simulink model "prob2_sim"  (R2013a)
settings: Solver=ode45  StartTime=0.0  StopTime=10.0  RelTol=1e-3
libraries: fl_lib x13, nesl_utility x7
settings Model: Creator=Suddenlink  LastModifiedBy=Suddenlink

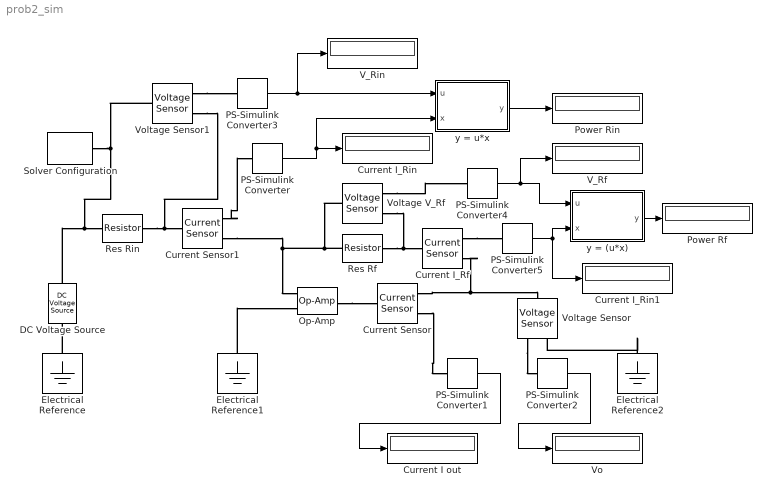
== system prob2_sim ==
  Current I out : Display
  Current I_Rf : fl_lib/Electrical/Electrical Sensors/Current Sensor  i1_Log=off  v1_Log=off  LocalVarNames=|i1|v1  LocalVarDescs=|i1|v1  LocalVarLogging=[0 0]
  Current I_Rin : Display
  Current I_Rin1 : Display
  Current Sensor : fl_lib/Electrical/Electrical Sensors/Current Sensor  i1_Log=off  v1_Log=off  LocalVarNames=|i1|v1  LocalVarDescs=|i1|v1  LocalVarLogging=[0 0]
  Current Sensor1 : fl_lib/Electrical/Electrical Sensors/Current Sensor  i1_Log=off  v1_Log=off  LocalVarNames=|i1|v1  LocalVarDescs=|i1|v1  LocalVarLogging=[0 0]
  DC Voltage Source : fl_lib/Electrical/Electrical Sources/DC Voltage Source  v0=5 V  i_Log=off  v_Log=off  LocalVarNames=|i|v  LocalVarDescs=|i|v  LocalVarLogging=[0 0]
  Electrical Reference : fl_lib/Electrical/Electrical Elements/Electrical Reference  i_Log=off  LocalVarNames=|i  LocalVarDescs=|i  LocalVarLogging=0
  Electrical Reference1 : fl_lib/Electrical/Electrical Elements/Electrical Reference  i_Log=off  LocalVarNames=|i  LocalVarDescs=|i  LocalVarLogging=0
  Electrical Reference2 : fl_lib/Electrical/Electrical Elements/Electrical Reference  i_Log=off  LocalVarNames=|i  LocalVarDescs=|i  LocalVarLogging=0
  Op-Amp : fl_lib/Electrical/Electrical Elements/Op-Amp  i1_Log=off  v1_Log=off  outI_Log=off  LocalVarNames=|i1|v1|outI  LocalVarDescs=|i1|v1|outI  LocalVarLogging=[0 0 0]
  PS-Simulink Converter{,1..5} (6 alike) : nesl_utility/PS-Simulink Converter  PhysicalDomain=network_engine_domain  SubClassName=ps_output  LeftPortType=input  RightPortType=output  PseudoPeriodic=off  Frequencies=[]  Unit=1  AffineConversion=off
  Power Rf : Display
  Power Rin : Display
  Res Rf : fl_lib/Electrical/Electrical Elements/Resistor  R=10000 Ohm  i_Log=off  v_Log=off  LocalVarNames=|i|v  LocalVarDescs=|i|v  LocalVarLogging=[0 0]
  "Res Rin " : fl_lib/Electrical/Electrical Elements/Resistor  R=1000 Ohm  i_Log=off  v_Log=off  LocalVarNames=|i|v  LocalVarDescs=|i|v  LocalVarLogging=[0 0]
  Solver Configuration : nesl_utility/Solver Configuration  PhysicalDomain=network_engine_domain  SubClassName=solver  LeftPortType=input  RightPortType=generic  Accelerate=off  Tones=[]  Harmonics=[]  SimulateNoise=off  Profile=off  UseLocalSampling=off  EnableSwitchedLinearOptims=on  FrequencyDomain=off  UseCCode=off  UseNewInitialization=off  DoDC=off  ResidualTolerance=1e-09  UseLocalSolver=off  LocalSolverChoice=NE_BACKWARD_EULER_ADVANCER  LocalSolverSampleTime=0.001  DoFixedCost=off  MaxNonlinIter=3  MaxModeIter=2  LinearAlgebra=Sparse  DelaysMemoryBudget=1024
  V_Rf : Display
  V_Rin : Display
  Vo : Display
  Voltage Sensor : fl_lib/Electrical/Electrical Sensors/Voltage Sensor  i1_Log=off  v1_Log=off  LocalVarNames=|i1|v1  LocalVarDescs=|i1|v1  LocalVarLogging=[0 0]
  Voltage Sensor1 : fl_lib/Electrical/Electrical Sensors/Voltage Sensor  i1_Log=off  v1_Log=off  LocalVarNames=|i1|v1  LocalVarDescs=|i1|v1  LocalVarLogging=[0 0]
  Voltage V_Rf : fl_lib/Electrical/Electrical Sensors/Voltage Sensor  i1_Log=off  v1_Log=off  LocalVarNames=|i1|v1  LocalVarDescs=|i1|v1  LocalVarLogging=[0 0]
  y = (u*x) : MATLAB Function  TreatAsAtomicUnit=on
  y = u*x : MATLAB Function  TreatAsAtomicUnit=on
  wires:
  PS-Simulink Converter/1 -> y = u*x/2(x), Current I_Rin/1
  PS-Simulink Converter1/1 -> Current I out/1
  PS-Simulink Converter2/1 -> Vo/1
  PS-Simulink Converter3/1 -> y = u*x/1(u), V_Rin/1
  y = u*x/1(y) -> Power Rin/1
  PS-Simulink Converter4/1 -> V_Rf/1, y = (u*x)/1(u)
  PS-Simulink Converter5/1 -> Current I_Rin1/1, y = (u*x)/2(x)
  y = (u*x)/1(y) -> Power Rf/1
  connections:
  Electrical Reference/LConn1 -- DC Voltage Source/RConn1
  DC Voltage Source/LConn1 -- Voltage Sensor1/LConn1 -- Solver Configuration/RConn1 -- "Res Rin "/LConn1
  "Res Rin "/RConn1 -- Voltage Sensor1/RConn2 -- Current Sensor1/LConn1
  Electrical Reference1/LConn1 -- Op-Amp/LConn2
  Op-Amp/RConn1 -- Current Sensor/LConn1
  Res Rf/LConn1 -- Voltage V_Rf/LConn1 -- Current Sensor1/RConn2 -- Op-Amp/LConn1
  Current Sensor/RConn2 -- Current I_Rf/RConn2 -- Voltage Sensor/LConn1
  Current Sensor1/RConn1 -- PS-Simulink Converter/LConn1
  Current Sensor/RConn1 -- PS-Simulink Converter1/LConn1
  Voltage Sensor/RConn1 -- PS-Simulink Converter2/LConn1
  Electrical Reference2/LConn1 -- Voltage Sensor/RConn2
  Voltage Sensor1/RConn1 -- PS-Simulink Converter3/LConn1
  Res Rf/RConn1 -- Voltage V_Rf/RConn2 -- Current I_Rf/LConn1
  Voltage V_Rf/RConn1 -- PS-Simulink Converter4/LConn1
  Current I_Rf/RConn1 -- PS-Simulink Converter5/LConn1

== matlab function prob2_sim/y = (u*x) ==
  data: u input; y output; x input
function y = fcn(u,x)
%#codegen

y = u*x;

== matlab function prob2_sim/y = u*x ==
  data: u input; y output; x input
function y = fcn(u,x)
%#codegen

y = u*x;
